simulink model "ECE411_Project_Student_Starter_baik2"  (R2022a)
settings: Solver=ode23tb  StartTime=0.0  StopTime=t_end  RelTol=1e-3
values from neighbouring files (symbols this model uses):
  Jm = 0.2    [ECE411_Project_Parameters_Starter.m]    (also in main_code.m = 0.02)
  Ki_wreg = Kp_wreg*(2*pi*1)    (= 37.6991118431)    [ECE411_Project_Parameters_Starter.m]    (also in main_code.m = 0.376991118431)
  Kp_wreg = Jm*30    (= 6)    [ECE411_Project_Parameters_Starter.m]    (also in main_code.m = 0.6)
  lambda_f = 0.0185    [ECE411_HW2_2_Parameters.m]    (also in main_code.m = lambda_f_RMS*sqrt(2))
  P = 8    [ECE411_HW2_2_Parameters.m]    (also in main_code.m)
  Te_cmd_max_neg = -20    [ECE411_Project_Parameters_Starter.m]    (also in main_code.m)
  Te_cmd_max_pos = 10    [ECE411_Project_Parameters_Starter.m]    (also in main_code.m)
  Te_test_part4a = -15    [ECE411_Project_Parameters_Starter.m]    (also in main_code.m)
  w_test_Part4a_RPM = 3000    [ECE411_Project_Parameters_Starter.m]    (also in main_code.m)
libraries: fl_lib x14, nesl_utility x14, ee_lib x3, eePwmGeneratorTwoLevel x1
settings Model: SimulationMode=accelerator  Creator=DiggerPC  LastModifiedBy=baikhyeongmeon
settings DebuggingCC: UnconnectedInputMsg=warning  UnconnectedOutputMsg=warning  UnconnectedLineMsg=warning
settings RTWCC: DLArmComputeVersion=19.05

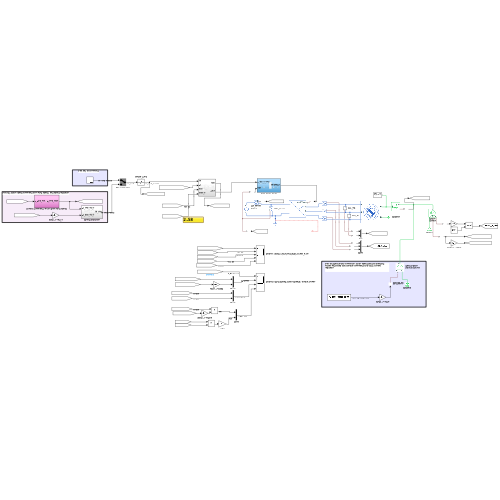
[thumbnail: Simulink's stored preview of the top-level diagram]
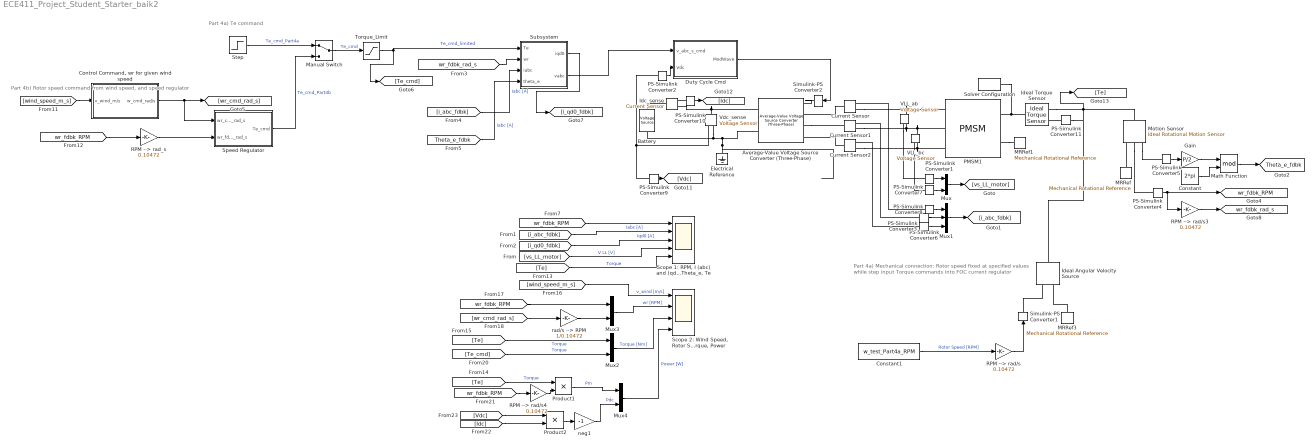
== system ECE411_Project_Student_Starter_baik2 ==
  note: Part 4a) Te command
  note: Part 4a) Mechanical connection: Rotor speed fixed at specified values while step input Torque commands into FOC current regulator
  note: Part 4b) Rotor speed command from wind speed, and speed regulator
  Average-Value Voltage Source Converter (Three-Phase) : ee_lib/Semiconductors & Converters/Converters/Average-Value Voltage Source Converter (Three-Phase)  port_option=ee.enum.threePhasePort.expanded  frequency_option=ee.enum.converters.frequency.variable  FRated=60 Hz  losses_parameterization=ee.enum.converters.losses.fixed  Pfixed=1 W  ks=0.01  kc1=1.7 V  kc2=0.01 Ohm  Ploss_vect=[100, 800, 1870, 3250, 4900] W  Irms_vect=[10, 100, 200, 300, 400] A  Vdc_nom=300 V  thermal_mass=30000 J/K  temperature_specify=off  temperature_priority=High  temperature=298.15 K  temperature_nominal_specify=off  temperature_nominal_unit=K  temperature_nominal_value=1
      settings: SourceProductBaseCode=PS  InternalSimscapePortConfiguration="{\"Bottom\":[],\"Left\":[{\"id\":\"ModWave\",\"label\":\"ModWave\",\"type\":\"input\"},{\"id\":\"a\",\"label\":\"a\",\"type\":\"foundation.electrical.electrical\"},{\"id\":\"b\",\"label\":\"b\",\"type\":\"foundation.electrical.electrical\"},{\"id\":\"c\",\"label\":\"c\",\"type\":\"foundation.electrical.electrical\"}],\"Right\":[{\"id\":\"p\",\"label\":\"+\",\"type\":\"foundation.electrical.electrical\"},{\"id\":\"n\",\"label\":\"-\",\"type\":\"foundation.electrical.electrical\"}],\"Top\":[]}"
  Battery : ee_lib/Sources/Voltage Source  dc_voltage=Vdc V  ac_voltage=0 V  ac_shift=0 rad  ac_frequency=60 Hz  noise_mode=0  PSD=0 V^2/Hz  repeatability=1  auto_seed=2249618129  user_seed=0  sample_time=1e-3 s  i_specify=off  i_priority=None  i=0 A  i_nominal_specify=off  i_nominal_unit=A  i_nominal_value=1  v_specify=off  v_priority=None  v=0 V  v_nominal_specify=off  v_nominal_unit=V  v_nominal_value=1
  Constant : Constant  Value=2*pi
  Constant1 : Constant  Value=w_test_Part4a_RPM
  "Control Command, wr for given wind speed" : Subsystem
  Current Sensor : fl_lib/Electrical/Electrical Sensors/Current Sensor
      settings: SourceProductBaseCode=PW,SS,VE
  Current Sensor1 : fl_lib/Electrical/Electrical Sensors/Current Sensor
      settings: SourceProductBaseCode=PW,SS,VE
  Current Sensor2 : fl_lib/Electrical/Electrical Sensors/Current Sensor
      settings: SourceProductBaseCode=PW,SS,VE
  Duty Cycle Cmd : Subsystem
  Electrical Reference : fl_lib/Electrical/Electrical Elements/Electrical Reference
      settings: SourceProductBaseCode=PW,SS,VE
  Gain : Gain  Gain=P/2
  Idc_sense : fl_lib/Electrical/Electrical Sensors/Current Sensor
      settings: SourceProductBaseCode=PW,SS,VE
  Ideal Angular Velocity Source : fl_lib/Mechanical/Mechanical Sources/Ideal Angular Velocity Source
      settings: SourceProductBaseCode=PW,SS,VE
  Ideal Torque Sensor : fl_lib/Mechanical/Mechanical Sensors/Ideal Torque Sensor
      settings: SourceProductBaseCode=PW,SS,VE
  MRRef : fl_lib/Mechanical/Rotational Elements/Mechanical Rotational Reference
      settings: SourceProductBaseCode=PW,SS,VE
  MRRef1 : fl_lib/Mechanical/Rotational Elements/Mechanical Rotational Reference
      settings: SourceProductBaseCode=PW,SS,VE
  MRRef3 : fl_lib/Mechanical/Rotational Elements/Mechanical Rotational Reference
      settings: SourceProductBaseCode=PW,SS,VE
  Manual Switch : ManualSwitch
  Math Function : Math  Operator=mod
  Motion Sensor : fl_lib/Mechanical/Mechanical Sensors/Ideal Rotational Motion Sensor  wrap_angle=simscape.enum.onoff.on  offset=0 deg
      settings: SourceProductBaseCode=PW,SS,VE
  Mux{,2..4} (4 alike) : Mux  Inputs=2
  Mux1 : Mux  Inputs=3
  PMSM1 : ee_lib/Electromechanical/Permanent Magnet/PMSM  port_option=ee.enum.threePhasePort.expanded  winding_type=ee.enum.statorconnection.wye  machine_param=ee.enum.pmsm.parameterization.constant  nPolePairs=P/2  pmflux_param=ee.enum.pmflux.fluxlinkage  pm_flux_linkage=lambda_f*sqrt(2) N*m/A  torque_constant=0.037*sqrt(2) N*m/A  back_emf_constant=0.037*sqrt(2) V/(rad/s)  stator_param=ee.enum.statorparam.LdLqL0  Ld=Lq H  Lq=Ld H  idVec=[-200, 0, 200] A  iqVec=[-200, 0, 200] A  LdMatrix=0.0002 * ones(3, 3) H  LqMatrix=0.0002 * ones(3, 3) H  PmMatrix=0.1 * ones(3, 3) Wb  ktMatrix=0.18 * ones(3, 3) N*m/A  keMatrix=0.18 * ones(3, 3) V/(rad/s)  L0=L0 H  Ls=Lqs H  Lm=0 H  Ms=0 H  Rs=Rs Ohm  zero_sequence=ee.enum.park.zerosequence.exclude  axes_param=ee.enum.rotorangle.qaxis  loss_param=ee.enum.ironloss.none  losses_oc=[0, 0, 0] W  losses_sc=[0, 0, 0] W  f_losses=60 Hz  Isc_losses=95 A  J=Jm kg*m^2  lam=0 N*m/(rad/s)  i_d_specify=off  i_d_priority=None  i_d=0 A  i_d_nominal_specify=off  i_d_nominal_unit=A  i_d_nominal_value=1  i_q_specify=off  i_q_priority=None  i_q=0 A  i_q_nominal_specify=off  i_q_nominal_unit=A  i_q_nominal_value=1  torque_specify=off  torque_priority=None  torque=0 N*m  torque_nominal_specify=off  torque_nominal_unit=N*m  torque_nominal_value=1  angular_velocity_specify=off  angular_velocity_priority=High  angular_velocity=0 rpm  angular_velocity_nominal_specify=off  angular_velocity_nominal_unit=rpm  angular_velocity_nominal_value=1  angular_position_specify=off  angular_position_priority=High  angular_position=0 deg  angular_position_nominal_specify=off  angular_position_nominal_unit=deg  angular_position_nominal_value=1  alpha=3.93e-3 1/K  alpha_flux=-0.001 1/K  Tmeas=298.15 K  stator_thermal_mass=100 J/K  rotor_thermal_mass=200 J/K  Rm_percent_rotor=90  Rd_percent_rotor=30  temperatureA_specify=off  temperatureA_priority=High  temperatureA=25 degC  temperatureA_nominal_specify=off  temperatureA_nominal_unit=degC  temperatureA_nominal_value=1  temperatureB_specify=off  temperatureB_priority=High  temperatureB=25 degC  temperatureB_nominal_specify=off  temperatureB_nominal_unit=degC  temperatureB_nominal_value=1  temperatureC_specify=off  temperatureC_priority=High  temperatureC=25 degC  temperatureC_nominal_specify=off  temperatureC_nominal_unit=degC  temperatureC_nominal_value=1  temperatureR_specify=off  temperatureR_priority=High  temperatureR=25 degC  temperatureR_nominal_specify=off  temperatureR_nominal_unit=degC  temperatureR_nominal_value=1
      settings: InternalSimscapePortConfiguration="{\"Bottom\":[],\"Left\":[{\"id\":\"a\",\"label\":\"a\",\"type\":\"foundation.electrical.electrical\"},{\"id\":\"b\",\"label\":\"b\",\"type\":\"foundation.electrical.electrical\"},{\"id\":\"c\",\"label\":\"c\",\"type\":\"foundation.electrical.electrical\"}],\"Right\":[{\"id\":\"R\",\"label\":\"R\",\"type\":\"foundation.mechanical.rotational.rotational\"},{\"id\":\"C\",\"label\":\"C\",\"type\":\"foundation.mechanical.rotational.rotational\"}],\"Top\":[]}"
  PS-Simulink Converter{1..2,7,9} (4 alike) : nesl_utility/PS-Simulink Converter  PhysicalDomain=network_engine_domain  SubClassName=ps_output  LeftPortType=input  RightPortType=output  PseudoPeriodic=off  Frequencies=[]  VectorFormat=1-D array  Unit=V  AffineConversion=off
      settings: SourceProductBaseCode=SS,PW,VE
  PS-Simulink Converter{3,6,8,10} (4 alike) : nesl_utility/PS-Simulink Converter  PhysicalDomain=network_engine_domain  SubClassName=ps_output  LeftPortType=input  RightPortType=output  PseudoPeriodic=off  Frequencies=[]  VectorFormat=1-D array  Unit=A  AffineConversion=off
      settings: SourceProductBaseCode=SS,PW,VE
  PS-Simulink Converter11 : nesl_utility/PS-Simulink Converter  PhysicalDomain=network_engine_domain  SubClassName=ps_output  LeftPortType=input  RightPortType=output  PseudoPeriodic=off  Frequencies=[]  VectorFormat=1-D array  Unit=N*m  AffineConversion=off
      settings: SourceProductBaseCode=SS,PW,VE
  PS-Simulink Converter4 : nesl_utility/PS-Simulink Converter  PhysicalDomain=network_engine_domain  SubClassName=ps_output  LeftPortType=input  RightPortType=output  PseudoPeriodic=off  Frequencies=[]  VectorFormat=1-D array  Unit=rpm  AffineConversion=off
      settings: SourceProductBaseCode=SS,PW,VE
  PS-Simulink Converter5 : nesl_utility/PS-Simulink Converter  PhysicalDomain=network_engine_domain  SubClassName=ps_output  LeftPortType=input  RightPortType=output  PseudoPeriodic=off  Frequencies=[]  VectorFormat=1-D array  Unit=rad  AffineConversion=off
      settings: SourceProductBaseCode=SS,PW,VE
  Product1 : Product  Inputs=**
  Product2 : Product  Inputs=**
  RPM --> rad/s : Gain  Gain=0.10472
  RPM --> rad/s3 : Gain  Gain=0.10472
  RPM --> rad/s4 : Gain  Gain=0.10472
  RPM --> rad_s : Gain  Gain=0.10472
  "Scope 1: RPM, I (abc) and (qd0), Theta_e, Te" : Scope  NumInputPorts=5
  "Scope 2: Wind Speed, Rotor Speeds, Torque, Power" : Scope  NumInputPorts=4
  Simulink-PS Converter1 : nesl_utility/Simulink-PS Converter  PhysicalDomain=network_engine_domain  SubClassName=ps_input  LeftPortType=input  RightPortType=output  PseudoPeriodic=off  Frequencies=[]  NoiseDistribution=none  NoiseParameters=[]  Unit=rad/s  AffineConversion=off  FilteringAndDerivatives=zero  SimscapeFilterOrder=1  InputFilterTimeConstant=0.001  UdotUserProvided=1
      settings: SourceProductBaseCode=SS,PW,VE
  Simulink-PS Converter2 : nesl_utility/Simulink-PS Converter  PhysicalDomain=network_engine_domain  SubClassName=ps_input  LeftPortType=input  RightPortType=output  PseudoPeriodic=off  Frequencies=[]  NoiseDistribution=none  NoiseParameters=[]  Unit=1  AffineConversion=off  FilteringAndDerivatives=provide  SimscapeFilterOrder=1  InputFilterTimeConstant=0.001  UdotUserProvided=0
      settings: SourceProductBaseCode=SS,PW,VE
  Solver Configuration : nesl_utility/Solver Configuration  PhysicalDomain=network_engine_domain  SubClassName=solver  LeftPortType=input  RightPortType=generic  Tones=[]  Harmonics=[]  SimulateNoise=off  Profile=off  UseLocalSampling=off  EnableSwitchedLinearOptims=on  FrequencyDomain=off  UseCCode=off  RelTol=0.001  AbsTol=1e-06  MinStep=1e-09  ToWorkspace=off  RevertToSquareIcSolve=off  NumHomotopyIterations=100  PhasorMode=off  PhasorModeNumHarmonics=1  IndexReductionMethod=DerivativeReplacement  DoDC=off  ResidualTolerance=1e-09  UseLocalSolver=on  LocalSolverChoice=NE_TRAPEZOIDAL_ADVANCER  LocalSolverSampleTime=1e-6  DoFixedCost=on  MaxNonlinIter=3  MaxModeIter=2  ComputeImpulses=off  ImpulseIterations=2  LinearAlgebra=auto  LinearAlgebraNumThread=0  EquationFormulation=NE_TIME_EF  DelaysMemoryBudget=1024  AutomaticFiltering=on  FilteringTimeConstant=0.001  PartitionStorageMethod=AS_NEEDED  PartitionMemoryBudget=1024  PartitionMethod=ROBUST
      settings: SourceProductBaseCode=SS,PW,VE
  Speed Regulator : Subsystem
  Step : Step  Time=0.1  After=Te_test_part4a  SampleTime=0
  Subsystem : Subsystem
  Torque_Limit : Saturate  UpperLimit=Te_cmd_max_pos  LowerLimit=Te_cmd_max_neg
  VLL_ab : fl_lib/Electrical/Electrical Sensors/Voltage Sensor
      settings: SourceProductBaseCode=PW,SS,VE
  VLL_bc : fl_lib/Electrical/Electrical Sensors/Voltage Sensor
      settings: SourceProductBaseCode=PW,SS,VE
  Vdc_sense : fl_lib/Electrical/Electrical Sensors/Voltage Sensor
      settings: SourceProductBaseCode=PW,SS,VE
  neg1 : Gain  Gain=-1
  rad/s --> RPM : Gain  Gain=1/0.10472
  tag scope: Theta_e_fdbk=global, wr_fdbk_RPM=global, wr_fdbk_rad_s=global
  wires:
  Mux/1 -> [vs_LL_motor]
  PS-Simulink Converter4/1 -> RPM --> rad/s3/1, [wr_fdbk_RPM]
  PS-Simulink Converter1/1 -> Mux/1
  PS-Simulink Converter5/1 -> Gain/1
  PS-Simulink Converter7/1 -> Mux/2
  [i_qd0_fdbk] -> "Scope 1: RPM, I (abc) and (qd0), Theta_e, Te"/3  "Iqd0 [A]"
  Gain/1 -> Math Function/1
  [i_abc_fdbk] -> "Scope 1: RPM, I (abc) and (qd0), Theta_e, Te"/2  "Iabc [A]"
  [vs_LL_motor] -> "Scope 1: RPM, I (abc) and (qd0), Theta_e, Te"/4  "V LL [V]"
  Math Function/1 -> [Theta_e_fdbk]
  Constant/1 -> Math Function/2
  PS-Simulink Converter2/1 -> Duty Cycle Cmd/2(Vdc)
  Duty Cycle Cmd/1(ModWave) -> Simulink-PS Converter2/1
  PS-Simulink Converter3/1 -> Mux1/3
  PS-Simulink Converter6/1 -> Mux1/2
  PS-Simulink Converter8/1 -> Mux1/1
  Mux1/1 -> [i_abc_fdbk]
  [wr_fdbk_RPM] -> "Scope 1: RPM, I (abc) and (qd0), Theta_e, Te"/1
  Manual Switch/1 -> Torque_Limit/1  "Te_cmd"
  Mux3/1 -> "Scope 2: Wind Speed, Rotor Speeds, Torque, Power"/2  "wr [RPM]"
  [wind_speed_m_s] -> "Scope 2: Wind Speed, Rotor Speeds, Torque, Power"/1  "v_wind [m/s]"
  RPM --> rad/s3/1 -> [wr_fdbk_rad_s]
  [wr_cmd_rad_s] -> rad/s --> RPM/1
  [Te] -> Mux2/1  "Torque"
  [Te_cmd] -> Mux2/2  "Torque"
  rad/s --> RPM/1 -> Mux3/2
  [wr_fdbk_RPM] -> Mux3/1
  Mux2/1 -> "Scope 2: Wind Speed, Rotor Speeds, Torque, Power"/3  "Torque [Nm]"
  PS-Simulink Converter9/1 -> [Vdc]
  PS-Simulink Converter10/1 -> [Idc]
  [wr_fdbk_RPM] -> RPM --> rad/s4/1
  RPM --> rad/s4/1 -> Product1/2
  [Te] -> Product1/1  "Torque"
  [Vdc] -> Product2/1
  [Idc] -> Product2/2
  Product1/1 -> Mux4/1  "Pm"
  Product2/1 -> neg1/1
  Mux4/1 -> "Scope 2: Wind Speed, Rotor Speeds, Torque, Power"/4  "Power [W]"
  neg1/1 -> Mux4/2  "Pdc"
  Constant1/1 -> RPM --> rad/s/1  "Rotor Speed [RPM]"
  RPM --> rad/s/1 -> Simulink-PS Converter1/1
  PS-Simulink Converter11/1 -> [Te]
  [Te] -> "Scope 1: RPM, I (abc) and (qd0), Theta_e, Te"/5  "Torque"
  [wr_fdbk_RPM] -> RPM --> rad_s/1
  "Control Command, wr for given wind speed"/1(w_cmd_rad/s) -> Speed Regulator/1(wr_cmd_rad_s), [wr_cmd_rad_s]
  Speed Regulator/1(Te_cmd) -> Manual Switch/2  "Te_cmd_Part4b"
  [wind_speed_m_s] -> "Control Command, wr for given wind speed"/1(v_wind_m/s)
  Step/1 -> Manual Switch/1  "Te_cmd_Part4a"
  RPM --> rad_s/1 -> Speed Regulator/2(wr_fdbk_rad_s)
  Torque_Limit/1 -> Subsystem/1(Te), [Te_cmd]  "Te_cmd_limited"
  Subsystem/2(vabc) -> Duty Cycle Cmd/1(v_abc_s_cmd)
  [wr_fdbk_rad_s] -> Subsystem/2(wr)
  Subsystem/1(iqd0) -> [i_qd0_fdbk]
  [i_abc_fdbk] -> Subsystem/3(iabc)  "Iabc [A]"
  [Theta_e_fdbk] -> Subsystem/4(theta_e)  "Iabc [A]"
  connections:
  Solver Configuration/RConn1 -- Ideal Torque Sensor/LConn1 -- PMSM1/RConn1
  VLL_ab/RConn1 -- PS-Simulink Converter1/LConn1
  Motion Sensor/RConn3 -- PS-Simulink Converter5/LConn1
  MRRef/LConn1 -- Motion Sensor/RConn1
  Motion Sensor/RConn2 -- PS-Simulink Converter4/LConn1
  PMSM1/RConn2 -- MRRef1/LConn1
  PS-Simulink Converter7/LConn1 -- VLL_bc/RConn1
  Electrical Reference/LConn1 -- Average-Value Voltage Source Converter (Three-Phase)/RConn2 -- Battery/RConn1 -- Vdc_sense/RConn2
  Vdc_sense/LConn1 -- Idc_sense/RConn2 -- Average-Value Voltage Source Converter (Three-Phase)/RConn1
  PS-Simulink Converter2/LConn1 -- Vdc_sense/RConn1 -- PS-Simulink Converter9/LConn1
  VLL_ab/LConn1 -- Current Sensor/RConn2 -- PMSM1/LConn1
  VLL_ab/RConn2 -- Current Sensor1/RConn2 -- PMSM1/LConn2 -- VLL_bc/LConn1
  VLL_bc/RConn2 -- Current Sensor2/RConn2 -- PMSM1/LConn3
  Current Sensor/LConn1 -- Average-Value Voltage Source Converter (Three-Phase)/LConn2
  Current Sensor2/LConn1 -- Average-Value Voltage Source Converter (Three-Phase)/LConn4
  Average-Value Voltage Source Converter (Three-Phase)/LConn3 -- Current Sensor1/LConn1
  PS-Simulink Converter3/LConn1 -- Current Sensor2/RConn1
  PS-Simulink Converter6/LConn1 -- Current Sensor1/RConn1
  PS-Simulink Converter8/LConn1 -- Current Sensor/RConn1
  Simulink-PS Converter2/RConn1 -- Average-Value Voltage Source Converter (Three-Phase)/LConn1
  Idc_sense/LConn1 -- Battery/LConn1
  Idc_sense/RConn1 -- PS-Simulink Converter10/LConn1
  Simulink-PS Converter1/RConn1 -- Ideal Angular Velocity Source/RConn1
  MRRef3/LConn1 -- Ideal Angular Velocity Source/RConn2
  Ideal Torque Sensor/RConn1 -- Motion Sensor/LConn1 -- Ideal Angular Velocity Source/LConn1
  PS-Simulink Converter11/LConn1 -- Ideal Torque Sensor/RConn2

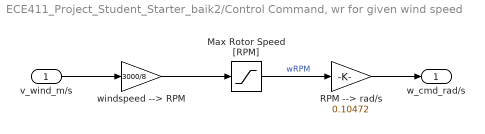
== system ECE411_Project_Student_Starter_baik2/Control Command, wr for given wind speed ==
  v_wind_m/s : Inport
  Max Rotor Speed [RPM] : Saturate  UpperLimit=3750  LowerLimit=0
  RPM --> rad/s : Gain  Gain=0.10472
  windspeed --> RPM : Gain  Gain=3000/8
  w_cmd_rad/s : Outport
  wires:
  v_wind_m/s/1 -> windspeed --> RPM/1
  Max Rotor Speed [RPM]/1 -> RPM --> rad/s/1  "wRPM"
  windspeed --> RPM/1 -> Max Rotor Speed [RPM]/1
  RPM --> rad/s/1 -> w_cmd_rad/s/1

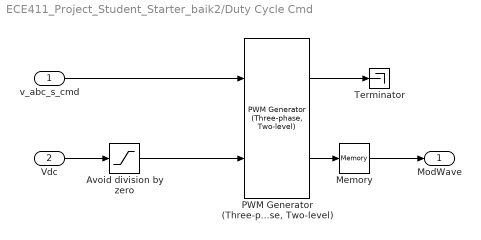
== system ECE411_Project_Student_Starter_baik2/Duty Cycle Cmd ==
  v_abc_s_cmd : Inport
  Vdc : Inport  Port=2
  Avoid division by zero : Saturate  UpperLimit=inf  LowerLimit=1
  Memory : Memory
  "PWM Generator (Three-phase, Two-level)" : eePwmGeneratorTwoLevel/PWM Generator (Three-phase, Two-level)  PWMMode=Continuous PWM (CPWM)  CPWMMode=SVM: space vector modulation  DPWMMode=60 DPWM: 60 degree discontinuous PWM  fsw=3000  Ts=1/30000
      settings: SourceProductBaseCode=PS
  Terminator : Terminator
  ModWave : Outport  VectorParamsAs1DForOutWhenUnconnected=off
  wires:
  Vdc/1 -> Avoid division by zero/1
  "PWM Generator (Three-phase, Two-level)"/2 -> Memory/1
  v_abc_s_cmd/1 -> "PWM Generator (Three-phase, Two-level)"/1
  Avoid division by zero/1 -> "PWM Generator (Three-phase, Two-level)"/2
  "PWM Generator (Three-phase, Two-level)"/1 -> Terminator/1
  Memory/1 -> ModWave/1

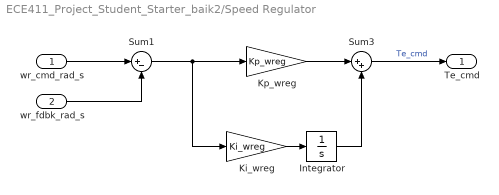
== system ECE411_Project_Student_Starter_baik2/Speed Regulator ==
  wr_cmd_rad_s : Inport
  wr_fdbk_rad_s : Inport  Port=2
  Integrator : Integrator
  Ki_wreg : Gain  Gain=Ki_wreg
  Kp_wreg : Gain  Gain=Kp_wreg
  Sum1 : Sum  Inputs=|+-
  Sum3 : Sum  Inputs=|++
  Te_cmd : Outport
  wires:
  Kp_wreg/1 -> Sum3/1
  Ki_wreg/1 -> Integrator/1
  Integrator/1 -> Sum3/2
  Sum1/1 -> Ki_wreg/1, Kp_wreg/1
  Sum3/1 -> Te_cmd/1  "Te_cmd"
  wr_fdbk_rad_s/1 -> Sum1/2
  wr_cmd_rad_s/1 -> Sum1/1

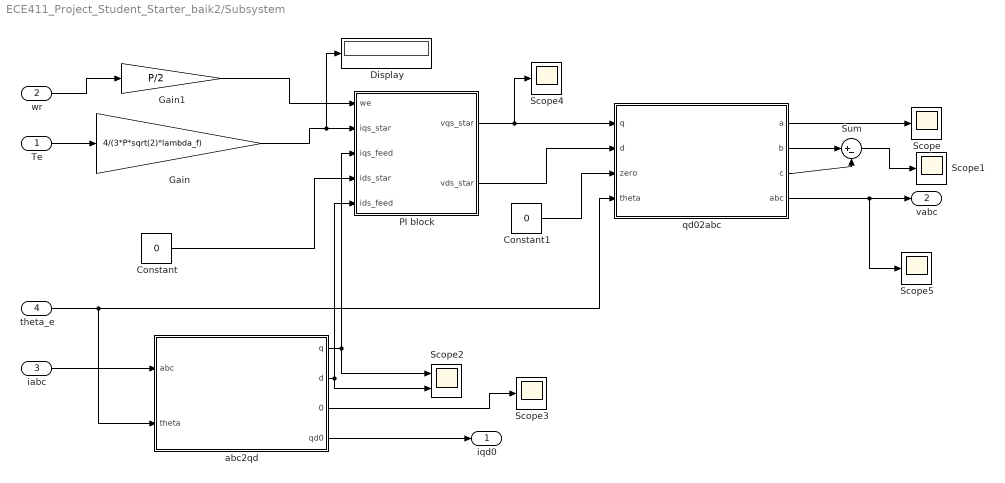
== system ECE411_Project_Student_Starter_baik2/Subsystem ==
  Te : Inport
  wr : Inport  Port=2
  iabc : Inport  Port=3
  theta_e : Inport  Port=4
  Constant : Constant  Value=0
  Constant1 : Constant  Value=0
  Display : Display
  Gain : Gain  Gain=4/(3*P*sqrt(2)*lambda_f)
  Gain1 : Gain  Gain=P/2
  PI block : Subsystem
  Scope{,1,3..5} (5 alike) : Scope
  Scope2 : Scope  NumInputPorts=2
  Sum : Sum  Inputs=|+-
  abc2qd : Subsystem
  qd02abc : Subsystem
  iqd0 : Outport
  vabc : Outport  Port=2
  wires:
  Te/1 -> Gain/1
  Gain/1 -> Display/1, PI block/2(iqs_star)
  Constant/1 -> PI block/4(ids_star)
  PI block/1(vqs_star) -> Scope4/1, qd02abc/1(q)
  PI block/2(vds_star) -> qd02abc/2(d)
  Constant1/1 -> qd02abc/3(zero)
  iabc/1 -> abc2qd/1(abc)
  abc2qd/4(qd0) -> iqd0/1
  abc2qd/1(q) -> Scope2/1, PI block/3(iqs_feed)
  abc2qd/2(d) -> Scope2/2, PI block/5(ids_feed)
  theta_e/1 -> abc2qd/2(theta), qd02abc/4(theta)
  wr/1 -> Gain1/1
  Gain1/1 -> PI block/1(we)
  qd02abc/1(a) -> Scope/1
  qd02abc/2(b) -> Sum/1
  qd02abc/3(c) -> Sum/2
  Sum/1 -> Scope1/1
  abc2qd/3(0) -> Scope3/1
  qd02abc/4(abc) -> Scope5/1, vabc/1

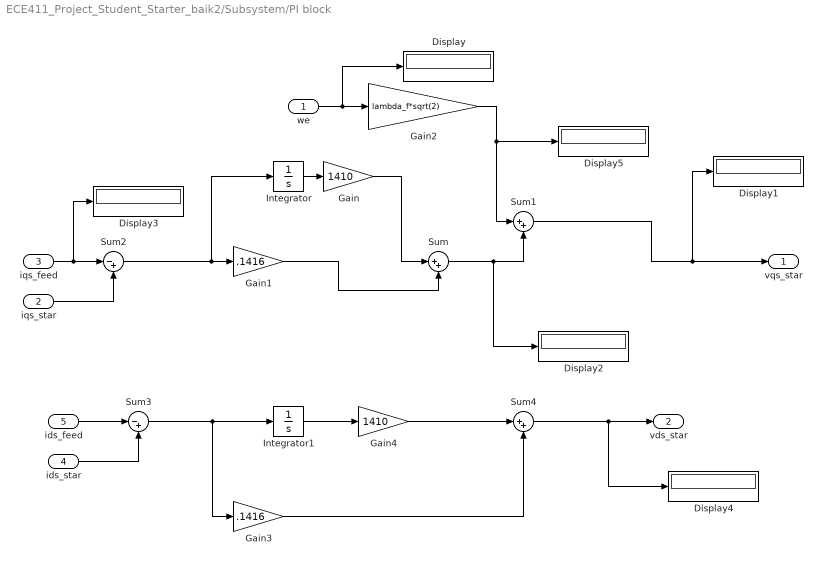
== system ECE411_Project_Student_Starter_baik2/Subsystem/PI block ==
  we : Inport
  iqs_star : Inport  Port=2
  iqs_feed : Inport  Port=3
  ids_star : Inport  Port=4
  ids_feed : Inport  Port=5
  Display{,1..5} (6 alike) : Display
  Gain : Gain  Gain=1410
  Gain1 : Gain  Gain=.1416
  Gain2 : Gain  Gain=lambda_f*sqrt(2)
  Gain3 : Gain  Gain=.1416
  Gain4 : Gain  Gain=1410
  Integrator : Integrator
  Integrator1 : Integrator
  Sum : Sum  Inputs=|++
  Sum1 : Sum  Inputs=|++
  Sum2 : Sum  Inputs=|-+
  Sum3 : Sum  Inputs=|-+
  Sum4 : Sum  Inputs=|++
  vqs_star : Outport
  vds_star : Outport  Port=2
  wires:
  Sum2/1 -> Integrator/1, Gain1/1
  Gain1/1 -> Sum/2
  Sum/1 -> Display2/1, Sum1/2
  Gain2/1 -> Sum1/1, Display5/1
  we/1 -> Display/1, Gain2/1
  Sum1/1 -> Display1/1, vqs_star/1
  Sum3/1 -> Integrator1/1, Gain3/1
  iqs_star/1 -> Sum2/2
  iqs_feed/1 -> Display3/1, Sum2/1
  ids_star/1 -> Sum3/2
  ids_feed/1 -> Sum3/1
  Gain3/1 -> Sum4/2
  Sum4/1 -> Display4/1, vds_star/1
  Integrator/1 -> Gain/1
  Gain/1 -> Sum/1
  Integrator1/1 -> Gain4/1
  Gain4/1 -> Sum4/1

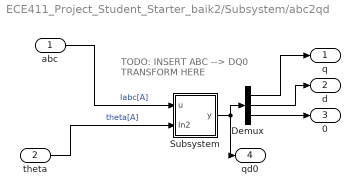
== system ECE411_Project_Student_Starter_baik2/Subsystem/abc2qd ==
  note: TODO: INSERT ABC --> DQ0 TRANSFORM HERE
  abc : Inport
  theta : Inport  Port=2
  Demux : Demux  Outputs=3
  Subsystem : Subsystem
  q : Outport
  d : Outport  Port=2
  0 : Outport  Port=3
  qd0 : Outport  Port=4
  wires:
  Demux/2 -> d/1
  theta/1 -> Subsystem/2(In2)  "theta[A]"
  Demux/1 -> q/1
  Subsystem/1(y) -> qd0/1, Demux/1
  Demux/3 -> 0/1
  abc/1 -> Subsystem/1(u)  "Iabc[A]"

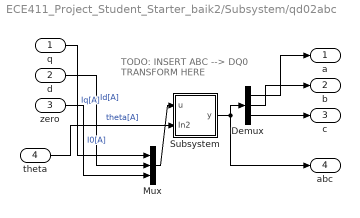
== system ECE411_Project_Student_Starter_baik2/Subsystem/qd02abc ==
  note: TODO: INSERT ABC --> DQ0 TRANSFORM HERE
  q : Inport
  d : Inport  Port=2
  zero : Inport  Port=3
  theta : Inport  Port=4
  Demux : Demux  Outputs=3
  Mux : Mux  Inputs=3
  Subsystem : Subsystem
  a : Outport
  b : Outport  Port=2
  c : Outport  Port=3
  abc : Outport  Port=4
  wires:
  Demux/2 -> b/1
  zero/1 -> Mux/3  "I0[A]"
  theta/1 -> Subsystem/2(In2)  "theta[A]"
  d/1 -> Mux/2  "Id[A]"
  q/1 -> Mux/1  "Iq[A]"
  Mux/1 -> Subsystem/1(u)
  Demux/1 -> a/1
  Subsystem/1(y) -> abc/1, Demux/1
  Demux/3 -> c/1

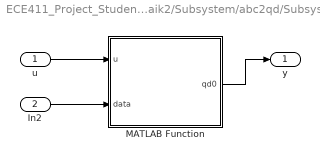
== system ECE411_Project_Student_Starter_baik2/Subsystem/abc2qd/Subsystem ==
  u : Inport
  In2 : Inport  Port=2
  MATLAB Function : MATLAB Function  TreatAsAtomicUnit=on
  y : Outport
  wires:
  u/1 -> MATLAB Function/1(u)
  In2/1 -> MATLAB Function/2(data)
  MATLAB Function/1(qd0) -> y/1

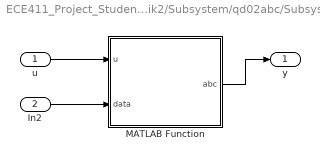
== system ECE411_Project_Student_Starter_baik2/Subsystem/qd02abc/Subsystem ==
  u : Inport
  In2 : Inport  Port=2
  MATLAB Function : MATLAB Function  TreatAsAtomicUnit=on
  y : Outport
  wires:
  u/1 -> MATLAB Function/1(u)
  In2/1 -> MATLAB Function/2(data)
  MATLAB Function/1(abc) -> y/1

== matlab function ECE411_Project_Student_Starter_baik2/Subsystem/qd02abc/Subsystem/MATLAB Function ==
  data: u input; abc output; data input
function abc = qd02alphabeta(u, data)

%% abc2alphabeta
T1 = 2/3*[1 -1/2 -1/2;0 -sqrt(3)/2 sqrt(3)/2; 1/sqrt(2) 1/sqrt(2) 1/sqrt(2)];
% alphabeta0= T1*u;

%% alphabeta2dq
T2_inv = [cos(data) sin(data) 0;-sin(data) cos(data) 0; 0 0 1];
alphabeta = T2_inv*u;

T1_inv = inv(T1);
abc = T1_inv*alphabeta;

end

== matlab function ECE411_Project_Student_Starter_baik2/Subsystem/abc2qd/Subsystem/MATLAB Function ==
  data: u input; qd0 output; data input
function qd0 = abc2qd0(u, data)

%% abc2alphabeta
T1 = 2/3*[1 -1/2 -1/2;0 -sqrt(3)/2 sqrt(3)/2; 1/2 1/2 1/2];
alphabeta0= T1*u;

%% alphabeta2qd
T2 = [cos(data) -sin(data) 0;sin(data) cos(data) 0; 0 0 1];
qd0 = T2*alphabeta0;



end
